simulink model "SimscapeCrane_MPChard"  (R2016a)
settings: Solver=ode15s  StartTime=0.0  StopTime=T  RelTol=1e-3
values from neighbouring files (symbols this model uses):
  bb = bbs(:, state) * 0.1    [MatlabSimulation.m]    (also in PartA_MPC.m = bbs(:,1); PartB.m = bbs(:,1); myTrajectoryConstraints.m = kron(ones(N, 1), bt); testMyMPC.m = bs)
  F = (DD * Gamma_tilda) + EE    [myConstraintMatrices.m]    (also in testMyMPC.m = Fs)
  G = 2 * Gamma' * Qbar * Phi    [myCostMatrices.m]
  H = 2 * (Rbar + Gamma' * Qbar * Gamma)    [myCostMatrices.m]    (also in testMyMPC.m = H\eye(size(H)); testMyMPC_soft.m = H\eye(size(H)))
  J = -(DD * Phi_tilda)    [myConstraintMatrices.m]    (also in testMyMPC.m = Js)
  L = - J - (DD * kron(ones(N, 1), eye(n)))    [myConstraintMatrices.m]    (also in testMyMPC.m = Ls)
  m = size(Gamma, 2)/N    [myConstraintMatrices.m]
  N = 10    [PartA.m]    (also in PartA_MPC.m = 20; PartA_RHC.m; PartB.m = 20; testMyMPC.m = ceil(Tf/Ts))
  stateMargin = [coordinateMargin, coordinateMargin, coordinateMargin, coordinateMargin, angleMargin, angleChangeMargin, angleMargin, angleChangeMargin]'    [PartA.m]    (also in PartA_MPC.m; PartA_RHC.m; PartB.m)
  Ts = 1/30    (= 0.0333333333333)    [PartA.m]    (also in PartA_MPC.m = 0.05; PartA_RHC.m; PartB.m = 0.05; testMyMPC.m = 0.1)
  X = responseRHC.output.signals.values(:,1)    [PartA_MPC.m]    (also in PartA_RHC.m; PartB.m)
  xTargets = [0.1, 0.1;              0.4, 0.1;              0.4, 0.4;              0.1, 0.4]    [PartA.m]    (also in PartA_MPC.m; PartA_RHC.m; PartB.m = [0.1, 0.1;              0.4, 0.1;              0.25, 0.4])
  xZero = xTargets(1,1)    [PartA_MPC.m]    (also in PartA_RHC.m = xRange(1); PartB.m; testMyMPC.m = xRange(1))
  Y = responseRHC.output.signals.values(:,3)    [PartA_MPC.m]    (also in PartA_RHC.m; PartB.m)
  yZero = xTargets(1,2)    [PartA_MPC.m]    (also in PartA_RHC.m = yRange(1); PartB.m; testMyMPC.m = yRange(1))
undefined symbols (not defined in the file or in its folder): MR, TxBreak, TxCoulomb, TxVisc, TyBreak, TyCoulomb, TzBreak, TzCoulomb, xRange, yRange, Z, zRange, zZero
undefined symbols (not defined in the file): M, TorqueMultX, TorqueMultY, TorqueMultZ, TxTrans, TyTrans, TyVisc, TzTrans, TzVisc
libraries: sm_lib x146, fl_lib x62, nesl_utility x24, elec_lib x9, simulink x6, sm_double_wishbone_suspension_lib x4, aerolibtransform2 x1
(part 1 of 14)
settings Model: Creator=jsustare  LastModifiedBy=acrisne
settings SolverCC: MaxConsecutiveMinStep=10
settings DataIOCC: SaveFormat=StructureWithTime
settings DebuggingCC: AllowSymbolicDim=off
settings ModelReferenceCC: PropagateSignalLabelsOutOfModel=off
settings GRTTargetCC: GeneratePreprocessorConditionals=Use local settings
settings ConfigurationSet: Description=SimMechanics 2G

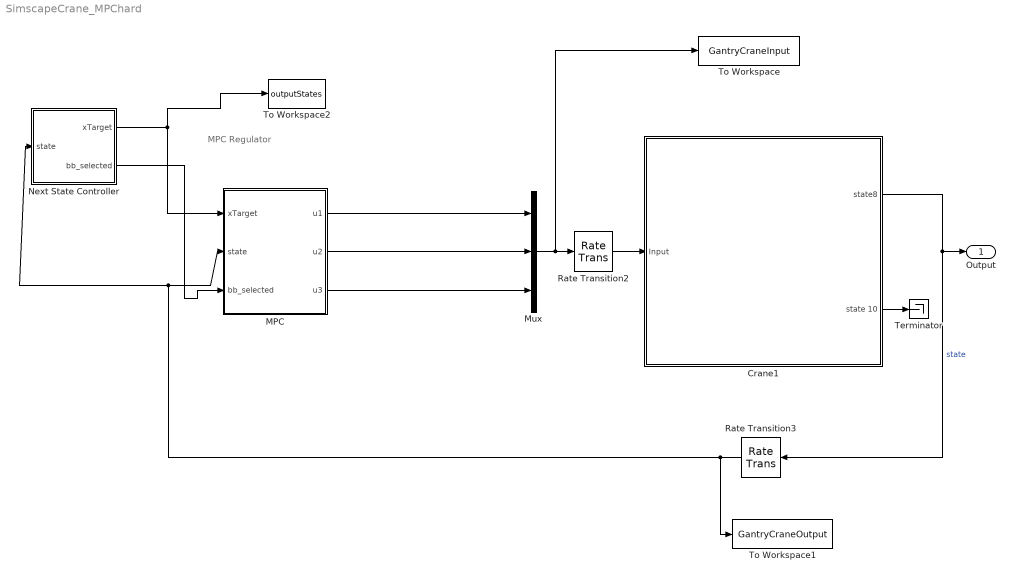
== system SimscapeCrane_MPChard ==
  note: MPC Regulator
  Crane1 : Subsystem  mask{penduMass=m, cartMass=M, MR=MR, xRange=xRange, yRange=yRange, zRange=zRange, xZero=xZero, yZero=yZero, zZero=zZero, TxBreak=TxBreak, TxCoulomb=TxCoulomb, TxVisc=TxVisc, TxTrans=TxTrans, TyBreak=TyBreak, TyCoulomb=TyCoulomb, TyVisc=TyVisc, TyTrans=TyTrans, TzBreak=TzBreak, TzCoulomb=TzCoulomb, TzVisc=TzVisc, TzTrans=TzTrans, Ux=TorqueMultX, Uy=TorqueMultY, Uz=TorqueMultZ}
      mask prompts: penduMass "Pendulum Mass (Kg)"; cartMass "Mass of the cart (Kg)"; MR "Mass of the rail (Kg)"; TxBreak "BreakAwayFriction"; TxCoulomb "Coulomb Friction"; TxVisc "Viscous friction"; TxTrans "Transition coeff"; TyBreak "BreakAwayFriction"; TyCoulomb "Coulomb Friction"; TyVisc "Viscous friction"; TyTrans "Transition coeff"; TzBreak "BreakAwayFriction"; TzCoulomb "Coulomb Friction"; TzVisc "Viscous friction"; TzTrans "Transition coeff"; Ux "Rail motor multiplier (X)"; Uy "Cart motor multiplier (Y)"; Uz "String motor multiplier (Z)"
      mask init:
      | %mass lowSat
      | penduMass=max(penduMass,1e-3);
      | cartMass=max(cartMass,1e-3);
      | MR=max(MR,1e-3);
      | 
      | %zeros saturated
      | xZero=max(xZero,xRange(1));
      | xZero=min(xZero,xRange(2));
      | 
      | yZero=max(yZero,yRange(1));
      | yZero=min(yZero,yRange(2));
      | 
      | zZero=max(zZero,zRange(1));
      | zZero=min(zZero,zRange(2));
      mask DialogControl DescGroupVar Prompt: 3D Crane Simscape model
      mask Display:
